simulink model "FM_Builtin"  (R2018b)
settings: Solver=VariableStepAuto  StartTime=0.0  StopTime=0.002  MaxStep=0.0000001  MinStep=0.000001  RelTol=1e-5
libraries: commanapbnd3 x3
settings Model: Creator=lenovo  LastModifiedBy=lenovo

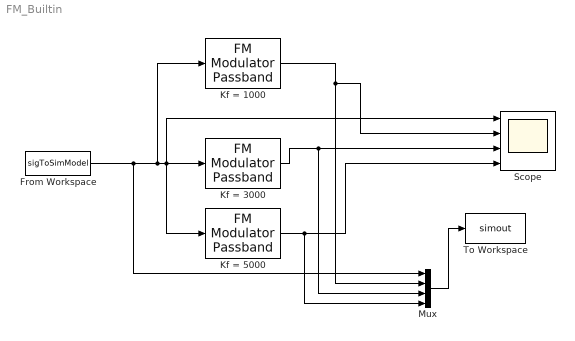
== system FM_Builtin ==
  From Workspace : FromWorkspace  VariableName=sigToSimModel  SampleTime=1e-7
  Kf = 1000 : commanapbnd3/FM Modulator Passband  Fc=10e3  Ph=0  Kc=1000
      settings: SourceProductName=Communications System Toolbox  SourceProductBaseCode=CM
  Kf = 3000 : commanapbnd3/FM Modulator Passband  Fc=10e3  Ph=0  Kc=3000
      settings: SourceProductName=Communications System Toolbox  SourceProductBaseCode=CM
  Kf = 5000 : commanapbnd3/FM Modulator Passband  Fc=10e3  Ph=0  Kc=5000
      settings: SourceProductName=Communications System Toolbox  SourceProductBaseCode=CM
  Mux : Mux
  Scope : Scope  NumInputPorts=4
  To Workspace : ToWorkspace  VariableName=simout  SaveFormat=Timeseries  SampleTime=-1
  wires:
  Kf = 5000/1 -> Mux/4, Scope/4
  Kf = 3000/1 -> Mux/3, Scope/3
  Kf = 1000/1 -> Mux/2, Scope/2
  From Workspace/1 -> Mux/1, Scope/1, Kf = 5000/1, Kf = 3000/1, Kf = 1000/1
  Mux/1 -> To Workspace/1
